simulink model "BD_HESS_K"  (R2024b)
settings: Solver=ode1  StartTime=0.0  StopTime=1369  FixedStep=0.1  MaxStep=1  RelTol=1e-3  AbsTol=1e-3
values from neighbouring files (symbols this model uses):
  ess2_cap = [ ... (first row only)    [ESS2_SC_MaxwellBCAP3400F.m]
  ess2_cap_scale = 1    [ESS2_SC_MaxwellBCAP3400F.m]
  ess2_coulombic_eff = [ ... (first row only)    [ESS2_SC_MaxwellBCAP3400F.m]
  ess2_init_soc = 1    [ESS2_SC_MaxwellBCAP3400F.m]
  ess2_max_volts = 2.7*120    (= 324)    [ESS2_SC_MaxwellBCAP3400F.m]
  ess2_min_volts = 0*2.7*120    (= 0)    [ESS2_SC_MaxwellBCAP3400F.m]
  ess2_mod_init_tmp = 20    [ESS2_SC_MaxwellBCAP3400F.m]
  ess2_module_num = 1    [ESS2_SC_MaxwellBCAP3400F.m]
  ess2_parallel_mod_num = 1    [ESS2_SC_MaxwellBCAP3400F.m]
  ess2_r = [ ... (first row only)    [ESS2_SC_MaxwellBCAP3400F.m]
  ess2_res_scale_coef = [1 0 1 0]    [ESS2_SC_MaxwellBCAP3400F.m]
  ess2_res_scale_fun = inline('(x(1)*ess2_module_num+x(2))/(x(3)*ess2_cap_scale+x(4))','x','ess2_module_num','ess2_cap_scale')    [ESS2_SC_MaxwellBCAP3400F.m]
  ess2_tmp = [-20 -10 0 5 10 15 20 25 30 40 50 60 65]    [ESS2_SC_MaxwellBCAP3400F.m]
  ess_cap_scale = 1    [ESS_Panasonic_NCR18650B_params.m]
  ess_coulombic_eff = [0.863 0.957 0.959 0.967 0.994]    [ESS_Panasonic_NCR18650B_params.m]
  ess_init_soc = 1    [ESS_Panasonic_NCR18650B_params.m]
  ess_max_ah_cap = [2.78 2.92 3.09 3.27 3.31]*74    [ESS_Panasonic_NCR18650B_params.m]
  ess_max_volts = 4.2*6    (= 25.2)    [ESS_Panasonic_NCR18650B_params.m]
  ess_min_volts = 2.5*6    (= 15)    [ESS_Panasonic_NCR18650B_params.m]
  ess_mod_init_tmp = 20    [ESS_Panasonic_NCR18650B_params.m]
  ess_module_num = 16    [ESS_Panasonic_NCR18650B_params.m]
  ess_on = 1    [ESS_Panasonic_NCR18650B_params.m]
  ess_r_chg = [0.0470 0.0457 0.0448 0.0435 0.0429 0.0427 0.0429 0.0462 ... (first row only)    [ESS_Panasonic_NCR18650B_params.m]
  ess_r_dis = [0.0470 0.0457 0.0448 0.0435 0.0429 0.0427 0.0429 0.0462 ... (first row only)    [ESS_Panasonic_NCR18650B_params.m]
  ess_res_scale_coef = [1 0 1 0]    [ESS_Panasonic_NCR18650B_params.m]
  ess_res_scale_fun = inline('(x(1)*ess_module_num+x(2))/(x(3)*ess_cap_scale+x(4))','x','ess_module_num','ess_cap_scale')    [ESS_Panasonic_NCR18650B_params.m]
  ess_soc = [0 10 20 40 60 80 90 100]/100    [ESS_Panasonic_NCR18650B_params.m]
  ess_tmp = [-10 0 10 25 45]    [ESS_Panasonic_NCR18650B_params.m]
  ess_voc = [2.5 2.74 2.93 3.17 3.36 3.5 3.49 3.34 ... (first row only)    [ESS_Panasonic_NCR18650B_params.m]
  mc_min_volts = 0    [ESS_Panasonic_NCR18650B_params.m]
  pth = pth_values(i)    [Ems_code_for_set_EMSvalue.m]
undefined symbols (not defined in the file or in its folder): power_load_in_Watt
(part 1 of 2)
settings Model: ModifiedComment=45089 -- Tue Apr 22 21:30:29 2025 -- Version 24.2  Creator=mokeefe  LastModifiedBy=ZULFI
settings Model: ModifiedHistory=|
  | 45089 -- Tue Apr 22 21:30:29 2025 -- Version 24.2
  | 
  | 45089 -- Tue Apr 22 21:18:21 2025 -- Version 24.1
  | 
  | 45089 -- Tue Apr 22 18:42:21 2025 -- Version 24.0
  | 
  | HP -- Sat Sep 19 16:11:01 2020 -- Version 1.240
  | 
  | 
  | HP -- Sat Sep 19 16:09:55 2020 -- Version 1.239
  | 
  | 
  | tz1n17 -- Sat Mar 30 21:57:00 2019 -- Version 1.238
  | 
  | 
  | tz1n17 -- Sat Mar 30 21:36:30 2019 -- Version 1.237
  | 
  | 
  | tz1n17 -- Sat Mar 30 21:35:16 2019 -- Version 1.236
  | 
  | 
  | tz1n17 -- Wed Mar 06 15:26:13 2019 -- Version 1.235
  | 
  | 
  | tz1n17 -- Wed Mar 06 15:22:09 2019 -- Version 1.234
  | 
  | 
  | tz1n17 -- Wed Mar 06 15:20:42 2019 -- Version 1.233
  | 
  | 
  | tz1n17 -- Wed Mar 06 15:19:06 2019 -- Version 1.232
  | 
  | 
  | tz1n17 -- Wed Mar 06 15:00:51 2019 -- Version 1.231
  | 
  | 
  | tz1n17 -- Wed Mar 06 14:47:09 2019 -- Version 1.230
  | 
  | 
  | tz1n17 -- Wed Mar 06 14:46:20 2019 -- Version 1.229
  | 
  | 
  | tz1n17 -- Wed Mar 06 14:42:10 2019 -- Version 1.228
  | 
  | 
  | tz1n17 -- Wed Mar 06 14:36:58 2019 -- Version 1.227
  | 
  | 
  | tz1n17 -- Wed Mar 06 13:46:14 2019 -- Version 1.226
  | 
  | 
  | tz1n17 -- Wed Mar 06 13:45:11 2019 -- Version 1.225
  | 
  | 
  | tz1n17 -- Wed Mar 06 12:23:18 2019 -- Version 1.224
  | 
  | 
  | tz1n17 -- Tue Mar 05 16:46:13 2019 -- Version 1.223
  | 
  | 
  | tz1n17 -- Tue Mar 05 16:36:09 2019 -- Version 1.222
  | 
  | 
  | tz1n17 -- Tue Mar 05 16:31:19 2019 -- Version 1.221
  | 
  | 
  | tz1n17 -- Tue Mar 05 15:30:42 2019 -- Version 1.220
  | 
  | 
  | tz1n17 -- Tue Mar 05 15:29:22 2019 -- Version 1.219
  | 
  | 
  | tz1n17 -- Tue Mar 05 15:24:15 2019 -- Version 1.218
  | 
  | 
  | tz1n17 -- Tue Mar 05 15:23:28 2019 -- Version 1.217
  | 
  | 
  | tz1n17 -- Tue Mar 05 15:23:21 2019 -- Version 1.216
  | 
  | 
  | tz1n17 -- Tue Mar 05 15:16:39 2019 -- Version 1.215
  | 
  | 
  | tz1n17 -- Tue Mar 05 15:14:45 2019 -- Version 1.214
  | 
  | 
  | tz1n17 -- Tue Mar 05 15:13:01 2019 -- Version 1.213
  | 
  | 
  | tz1n17 -- Tue Mar 05 15:09:24 2019 -- Version 1.212
  | 
  | 
  | tz1n17 -- Tue Mar 05 15:02:33 2019 -- Version 1.211
  | 
  | 
  | tz1n17 -- Tue Mar 05 15:01:02 2019 -- Version 1.210
  | 
  | 
  | tz1n17 -- Mon Mar 04 22:33:33 2019 -- Version 1.209
  | 
  | 
  | tz1n17 -- Mon Mar 04 22:09:23 2019 -- Version 1.208
  | 
  | 
  | tz1n17 -- Mon Mar 04 21:44:15 2019 -- Version 1.207
  | 
  | 
  | tz1n17 -- Mon Mar 04 21:41:50 2019 -- Version 1.206
  | 
  | 
  | tz1n17 -- Mon Mar 04 21:41:07 2019 -- Version 1.205
  | 
  | 
  | HP -- Mon Mar 04 01:45:44 2019 -- Version 1.204
  | 
  | 
  | HP -- Mon Mar 04 01:39:57 2019 -- Version 1.203
  | 
  | 
  | HP -- Mon Mar 04 01:37:38 2019 -- Version 1.202
  | 
  | 
  | HP -- Mon Mar 04 01:08:49 2019 -- Version 1.201
  | 
  | 
  | HP -- Mon Mar 04 01:02:45 2019 -- Version 1.200
  | 
  | 
  | HP -- Mon Mar 04 00:48:56 2019 -- Version 1.199
  | 
  | 
  | tz1n17 -- Sun Mar 03 22:48:13 2019 -- Version 1.198
  | 
  | 
  | tz1n17 -- Sun Mar 03 22:46:29 2019 -- Version 1.197
  | 
  | 
  | tz1n17 -- Sun Mar 03 21:57:47 2019 -- Version 1.196
  | 
  | 
  | tz1n17 -- Sun Mar 03 21:10:24 2019 -- Version 1.195
  | 
  | 
  | tz1n17 -- Sun Mar 03 21:06:11 2019 -- Version 1.194
  | 
  | 
  | tz1n17 -- Sun Mar 03 20:55:37 2019 -- Version 1.193
  | 
  | 
  | tz1n17 -- Sun Mar 03 20:49:58 2019 -- Version 1.192
  | 
  | 
  | tz1n17 -- Mon Feb 25 15:47:07 2019 -- Version 1.191
  | 
  | 
  | tz1n17 -- Mon Feb 25 15:37:36 2019 -- Version 1.190
  | 
  | 
  | tz1n17 -- Mon Feb 25 14:55:26 2019 -- Version 1.189
  | 
  | 
  | tz1n17 -- Mon Feb 25 14:54:22 2019 -- Version 1.188
  | 
  | 
  | tz1n17 -- Mon Feb 25 14:54:08 2019 -- Version 1.187
  | 
  | 
  | tz1n17 -- Fri Feb 15 22:56:00 2019 -- Version 1.186
  | 
  | 
  | tz1n17 -- Wed Dec 19 14:48:50 2018 -- Version 1.185
  | 
  | 
  | tz1n17 -- Tue Dec 18 22:44:41 2018 -- Version 1.184
  | 
  | 
  | tz1n17 -- Tue Dec 18 18:15:37 2018 -- Version 1.183
  | 
  | 
  | tz1n17 -- Tue Dec 18 18:08:38 2018 -- Version 1.182
  | 
  | 
  | tz1n17 -- Tue Dec 18 17:38:08 2018 -- Version 1.181
  | 
  | 
  | tz1n17 -- Mon Dec 17 22:41:01 2018 -- Version 1.180
  | 
  | 
  | tz1n17 -- Mon Dec 17 20:34:34 2018 -- Version 1.179
  | 
  | 
  | tz1n17 -- Mon Dec 17 17:22:02 2018 -- Version 1.178
  | 
  | 
  | tz1n17 -- Wed Dec 12 22:54:23 2018 -- Version 1.177
  | 
  | 
  | tz1n17 -- Wed Dec 12 20:45:31 2018 -- Version 1.176
  | 
  | 
  | tz1n17 -- Tue Dec 11 15:05:18 2018 -- Version 1.175
  | 
  | 
  | tz1n17 -- Tue Dec 11 14:54:48 2018 -- Version 1.174
  | 
  | 
  | tz1n17 -- Tue Dec 11 14:50:01 2018 -- Version 1.173
  | 
  | 
  | tz1n17 -- Tue Dec 11 14:47:20 2018 -- Version 1.172
  | 
  | 
  | tz1n17 -- Tue Dec 11 14:46:21 2018 -- Version 1.171
  | 
  | 
  | tz1n17 -- Tue Dec 11 14:36:41 2018 -- Version 1.170
  | 
  | 
  | tz1n17 -- Tue Dec 11 14:22:13 2018 -- Version 1.169
  | 
  | 
  | tz1n17 -- Tue Dec 11 14:20:14 2018 -- Version 1.168
  | 
  | 
  | tz1n17 -- Sun Dec 09 22:34:26 2018 -- Version 1.167
  | 
  | 
  | tz1n17 -- Sun Dec 09 22:33:45 2018 -- Version 1.166
  | 
  | 
  | tz1n17 -- Sun Dec 09 22:25:11 2018 -- Version 1.165
  | 
  | 
  | tz1n17 -- Sun Dec 09 22:23:19 2018 -- Version 1.164
  | 
  | 
  | tz1n17 -- Sun Dec 09 22:22:45 2018 -- Version 1.163
  | 
  | 
  | tz1n17 -- Sun Dec 09 22:21:43 2018 -- Version 1.162
  | 
  | 
  | tz1n17 -- Sun Dec 09 22:20:11 2018 -- Version 1.161
  | 
  | 
  | tz1n17 -- Sun Dec 09 22:19:52 2018 -- Version 1.160
  | 
  | 
  | tz1n17 -- Sun Dec 09 22:01:56 2018 -- Version 1.159
  | 
  | 
  | tz1n17 -- Sun Dec 09 21:58:21 2018 -- Version 1.158
  | 
  | 
  | tz1n17 -- Sun Dec 09 21:55:12 2018 -- Version 1.157
  | 
  | 
  | tz1n17 -- Sun Dec 09 21:51:49 2018 -- Version 1.156
  | 
  | 
  | tz1n17 -- Sun Dec 09 21:49:03 2018 -- Version 1.155
  | 
  | 
  | tz1n17 -- Sun Dec 09 21:48:14 2018 -- Version 1.154
  | 
  | 
  | tz1n17 -- Sun Dec 09 21:32:48 2018 -- Version 1.153
  | 
  | 
  | tz1n17 -- Sun Dec 09 20:07:47 2018 -- Version 1.152
  | 
  | 
  | tz1n17 -- Sun Dec 09 18:47:48 2018 -- Version 1.151
  | 
  | 
  | tz1n17 -- Sun Dec 09 18:18:43 2018 -- Version 1.150
  | 
  | 
  | HP -- Sun Dec 09 02:13:19 2018 -- Version 1.149
  | 
  | 
  | tz1n17 -- Sat Dec 08 22:45:48 2018 -- Version 1.148
  | 
  | 
  | tz1n17 -- Sat Dec 08 18:27:05 2018 -- Version 1.147
  | 
  | 
  | HP -- Sat Dec 08 00:10:24 2018 -- Version 1.146
  | 
  | 
  | HP -- Sat Dec 08 00:03:06 2018 -- Version 1.145
  | 
  | 
  | HP -- Fri Dec 07 23:56:35 2018 -- Version 1.144
  | 
  | 
  | tz1n17 -- Fri Dec 07 22:43:57 2018 -- Version 1.143
  | 
  | 
  | tz1n17 -- Fri Dec 07 22:21:30 2018 -- Version 1.142
  | 
  | 
  | tz1n17 -- Fri Dec 07 21:44:41 2018 -- Version 1.141
  | 
  | 
  | tz1n17 -- Fri Dec 07 21:41:03 2018 -- Version 1.140
  | 
  | 
  | tz1n17 -- Fri Dec 07 21:39:48 2018 -- Version 1.139
  | 
  | 
  | tz1n17 -- Fri Dec 07 18:02:33 2018 -- Version 1.138
  | 
  | 
  | tz1n17 -- Fri Dec 07 17:48:39 2018 -- Version 1.137
  | 
  | 
  | tz1n17 -- Fri Dec 07 15:16:04 2018 -- Version 1.136
  | 
  | 
  | tz1n17 -- Fri Dec 07 15:05:37 2018 -- Version 1.135
  | 
  | 
  | tz1n17 -- Fri Dec 07 14:56:20 2018 -- Version 1.134
  | 
  | 
  | tz1n17 -- Fri Dec 07 13:49:20 2018 -- Version 1.133
  | 
  | 
  | tz1n17 -- Fri Dec 07 13:47:15 2018 -- Version 1.132
  | 
  | 
  | tz1n17 -- Thu Dec 06 15:55:35 2018 -- Version 1.131
  | 
  | 
  | tz1n17 -- Thu Dec 06 15:03:27 2018 -- Version 1.130
  | 
  | 
  | tz1n17 -- Tue Dec 04 17:57:34 2018 -- Version 1.129
  | 
  | 
  | tz1n17 -- Tue Dec 04 15:03:13 2018 -- Version 1.128
  | 
  | 
  | tz1n17 -- Tue Dec 04 14:53:19 2018 -- Version 1.127
  | 
  | 
  | tz1n17 -- Tue Dec 04 14:45:06 2018 -- Version 1.126
  | 
  | 
  | tz1n17 -- Tue Dec 04 14:39:30 2018 -- Version 1.125
  | 
  | 
  | tz1n17 -- Tue Dec 04 14:29:06 2018 -- Version 1.124
  | 
  | 
  | HP -- Sun Dec 02 02:48:45 2018 -- Version 1.123
  | 
  | 
  | HP -- Sun Dec 02 01:47:26 2018 -- Version 1.122
  | 
  | 
  | HP -- Sun Dec 02 01:13:09 2018 -- Version 1.121
  | 
  | 
  | tz1n17 -- Sat Dec 01 23:02:41 2018 -- Version 1.120
  | 
  | 
  | tz1n17 -- Sat Dec 01 23:01:08 2018 -- Version 1.119
  | 
  | 
  | tz1n17 -- Sat Dec 01 22:57:45 2018 -- Version 1.118
  | 
  | 
  | tz1n17 -- Wed Nov 28 20:22:41 2018 -- Version 1.117
  | 
  | 
  | tz1n17 -- Wed Nov 28 20:01:59 2018 -- Version 1.116
  | 
  | 
  | tz1n17 -- Wed Nov 28 20:00:05 2018 -- Version 1.115
  | 
  | 
  | tz1n17 -- Wed Nov 28 19:59:42 2018 -- Version 1.114
  | 
  | 
  | tz1n17 -- Wed Nov 28 19:39:22 2018 -- Version 1.113
  | 
  | 
  | tz1n17 -- Wed Nov 28 19:29:55 2018 -- Version 1.112
  | 
  | 
  | tz1n17 -- Wed Nov 28 19:29:15 2018 -- Version 1.111
  | 
  | 
  | tz1n17 -- Wed Nov 28 19:28:44 2018 -- Version 1.110
  | 
  | 
  | tz1n17 -- Wed Nov 28 19:26:40 2018 -- Version 1.109
  | 
  | 
  | tz1n17 -- Wed Nov 28 19:25:31 2018 -- Version 1.108
  | 
  | 
  | tz1n17 -- Wed Nov 28 19:24:33 2018 -- Version 1.107
  | 
  | 
  | tz1n17 -- Wed Nov 28 19:15:20 2018 -- Version 1.106
  | 
  | 
  | tz1n17 -- Wed Nov 28 19:13:31 2018 -- Version 1.105
  | 
  | 
  | tz1n17 -- Wed Nov 28 19:11:29 2018 -- Version 1.103
  | 
  | 
  | tz1n17 -- Wed Nov 28 19:12:22 2018 -- Version 1.103
  | 
  | 
  | tz1n17 -- Wed Nov 28 19:08:22 2018 -- Version 1.102
  | 
  | 
  | tz1n17 -- Wed Nov 28 19:03:07 2018 -- Version 1.101
  | 
  | 
  | tz1n17 -- Wed Nov 28 18:47:53 2018 -- Version 1.100
  | 
  | 
  | tz1n17 -- Wed Nov 28 18:45:05 2018 -- Version 1.99
  | 
  | 
  | tz1n17 -- Wed Nov 28 18:29:30 2018 -- Version 1.98
  | 
  | 
  | tz1n17 -- Wed Nov 28 18:02:53 2018 -- Version 1.97
  | 
  | 
  | tz1n17 -- Wed Nov 28 18:01:36 2018 -- Version 1.96
  | 
  | 
  | tz1n17 -- Wed Nov 28 17:50:17 2018 -- Version 1.95
  | 
  | 
  | tz1n17 -- Wed Nov 28 17:44:30 2018 -- Version 1.94
  | 
  | 
  | tz1n17 -- Wed Nov 28 17:38:14 2018 -- Version 1.93
  | 
  | 
  | tz1n17 -- Wed Nov 28 15:16:29 2018 -- Version 1.92
  | 
  | 
  | tz1n17 -- Wed Nov 28 15:15:00 2018 -- Version 1.91
  | 
  | 
  | tz1n17 -- Wed Nov 28 15:13:10 2018 -- Version 1.90
  | 
  | 
  | tz1n17 -- Wed Nov 28 15:12:41 2018 -- Version 1.89
  | 
  | 
  | tz1n17 -- Wed Nov 28 15:10:02 2018 -- Version 1.88
  | 
  | 
  | tz1n17 -- Wed Nov 28 15:05:39 2018 -- Version 1.87
  | 
  | 
  | tz1n17 -- Wed Nov 28 15:05:01 2018 -- Version 1.86
  | 
  | 
  | tz1n17 -- Wed Nov 28 14:59:02 2018 -- Version 1.85
  | 
  | 
  | tz1n17 -- Wed Nov 28 14:58:38 2018 -- Version 1.84
  | 
  | 
  | tz1n17 -- Wed Nov 28 14:57:57 2018 -- Version 1.83
  | 
  | 
  | tz1n17 -- Wed Nov 28 14:56:25 2018 -- Version 1.82
  | 
  | 
  | tz1n17 -- Wed Nov 28 14:55:58 2018 -- Version 1.81
  | 
  | 
  | tz1n17 -- Wed Nov 28 14:54:44 2018 -- Version 1.80
  | 
  | 
  | tz1n17 -- Wed Nov 28 14:52:16 2018 -- Version 1.79
  | 
  | 
  | tz1n17 -- Wed Nov 28 14:50:51 2018 -- Version 1.78
  | 
  | 
  | tz1n17 -- Wed Nov 28 14:50:00 2018 -- Version 1.77
  | 
  | 
  | tz1n17 -- Wed Nov 28 14:45:14 2018 -- Version 1.76
  | 
  | 
  | tz1n17 -- Wed Nov 28 14:33:34 2018 -- Version 1.75
  | 
  | 
  | tz1n17 -- Wed Nov 28 13:43:19 2018 -- Version 1.74
  | 
  | 
  | tz1n17 -- Tue Nov 27 23:20:40 2018 -- Version 1.73
  | 
  | 
  | tz1n17 -- Tue Nov 27 23:12:46 2018 -- Version 1.72
  | 
  | 
  | tz1n17 -- Tue Nov 27 23:10:27 2018 -- Version 1.71
  | 
  | 
  | tz1n17 -- Tue Nov 27 20:21:58 2018 -- Version 1.70
  | 
  | 
  | tz1n17 -- Tue Nov 27 20:17:34 2018 -- Version 1.69
  | 
  | 
  | tz1n17 -- Tue Nov 27 20:09:17 2018 -- Version 1.68
  | 
  | 
  | tz1n17 -- Tue Nov 27 20:06:13 2018 -- Version 1.67
  | 
  | 
  | tz1n17 -- Tue Nov 27 19:10:28 2018 -- Version 1.66
  | 
  | 
  | tz1n17 -- Tue Nov 27 18:48:36 2018 -- Version 1.65
  | 
  | 
  | tz1n17 -- Tue Nov 27 18:42:18 2018 -- Version 1.64
  | 
  | 
  | tz1n17 -- Tue Nov 27 18:22:46 2018 -- Version 1.63
  | 
  | 
  | tz1n17 -- Tue Nov 27 18:11:41 2018 -- Version 1.62
  | 
  | 
  | tz1n17 -- Tue Nov 27 17:00:22 2018 -- Version 1.61
  | 
  | 
  | tz1n17 -- Tue Nov 27 16:46:06 2018 -- Version 1.60
  | 
  | 
  | tz1n17 -- Tue Nov 27 16:40:59 2018 -- Version 1.59
  | 
  | 
  | tz1n17 -- Tue Nov 27 14:28:49 2018 -- Version 1.58
  | 
  | 
  | tz1n17 -- Tue Nov 27 14:23:14 2018 -- Version 1.57
  | 
  | 
  | tz1n17 -- Tue Nov 27 14:01:43 2018 -- Version 1.56
  | 
  | 
  | tz1n17 -- Tue Nov 27 14:01:03 2018 -- Version 1.55
  | 
  | 
  | tz1n17 -- Tue Nov 27 13:50:04 2018 -- Version 1.54
  | 
  | 
  | tz1n17 -- Tue Nov 27 13:39:43 2018 -- Version 1.53
  | 
  | 
  | tz1n17 -- Mon Nov 26 22:49:44 2018 -- Version 1.52
  | 
  | 
  | tz1n17 -- Mon Nov 26 21:02:43 2018 -- Version 1.51
  | 
  | 
  | tz1n17 -- Mon Nov 26 20:38:16 2018 -- Version 1.50
  | 
  | 
  | tz1n17 -- Mon Nov 26 14:59:15 2018 -- Version 1.49
  | 
  | 
  | tz1n17 -- Mon Nov 26 14:25:02 2018 -- Version 1.48
  | 
  | 
  | tz1n17 -- Sun Nov 25 17:04:50 2018 -- Version 1.47
  | 
  | 
  | tz1n17 -- Sun Nov 25 16:33:53 2018 -- Version 1.46
  | 
  | 
  | tz1n17 -- Sat Nov 24 23:14:29 2018 -- Version 1.45
  | 
  | 
  | tz1n17 -- Wed Nov 21 22:02:06 2018 -- Version 1.44
  | 
  | 
  | tz1n17 -- Mon Oct 29 23:01:38 2018 -- Version 1.43
  | 
  | 
  | tz1n17 -- Mon Oct 29 22:46:10 2018 -- Version 1.42
  | 
  | 
  | tz1n17 -- Mon Oct 29 22:41:06 2018 -- Version 1.41
  | 
  | 
  | tz1n17 -- Mon Oct 29 22:23:29 2018 -- Version 1.40
  | 
  | 
  | tz1n17 -- Mon Oct 29 16:17:50 2018 -- Version 1.39
  | 
  | 
  | mokeefe -- Fri Mar 23 15:18:43 2012 -- Version 1.38
  | Updated parameterized link to restore library link. Save to update to newset Simulink version.
  | 
  | ssprik -- Wed Sep 24 14:52:29 2003 -- Version 1.37
  | 
  | 
  | abrooker -- Tue May 14 11:43:34 2002 -- Version 1.36
  | 
  | 
  | mokeefe -- Thu Apr 18 07:55:22 2002 -- Version 1.35
  | saving the model:
  | o "without the model browser open"
  | o with only top-level screen visible
  | o and with "fit to view" enabled
  | 
  | mokeefe -- Thu Apr 18 07:44:56 2002 -- Version 1.34
  | saving the model:
  | o "without the model browser open"
  | o with only top-level screen visible
  | o and with "fit to view" enabled
settings SolverCC: AutoScaleAbsTol=off  AlgebraicLoopSolver=TrustRegion
settings DataIOCC: SaveFormat=Array  SignalLoggingSaveFormat=ModelDataLogs  SaveOutput=off  SaveTime=off  ReturnWorkspaceOutputs=off
settings OptimizationCC: BooleanDataType=off  ExpressionDepthLimit=2147483647  LifeSpan=inf
settings DebuggingCC: SaveWithParameterizedLinksMsg=none  UnderspecifiedInitializationDetection=Classic  MergeDetectMultiDrivingBlocksExec=none  SignalResolutionControl=TryResolveAllWithWarning  MultiTaskDSMMsg=warning  MultiTaskCondExecSysMsg=none  FcnCallInpInsideContextMsg=warning  UnconnectedInputMsg=warning  UnconnectedOutputMsg=warning  StateNameClashWarn=warning  SFUnexpectedBacktrackingDiag=warning  SFNoUnconditionalDefaultTransitionDiag=warning  SFExecutionAtInitializationDiag=none  ArithmeticOperatorsInVariantConditions=warning
settings HardwareCC: ProdBitPerPointer=32  ProdBitPerSizeT=32  ProdBitPerPtrDiffT=32  ProdLargestAtomicFloat=None  ProdIntDivRoundTo=Undefined  ProdEndianess=Unspecified  ProdWordSize=32  ProdHWDeviceType=32-bit Generic  TargetUnknown=on
settings ModelReferenceCC: PropagateSignalLabelsOutOfModel=off
settings SFSimCC: SimUseLocalCustomCode=off  CustomCodeUndefinedFunction=UseInterfaceOnly
settings RTWCC: TemplateMakefile=grt_vc.tmf  RTWUseLocalCustomCode=off  GPUComputeCapability=3.5
settings CodeAppCC: StateflowObjectComments=on
settings GRTTargetCC: TargetLangStandard=C89/C90 (ANSI)  CombineOutputUpdateFcns=off  GRTInterface=on
settings ConfigComp: CovMetricSettings=dw  CovSaveCumulativeToWorkspaceVar=on  CovSaveSingleToWorkspaceVar=on  CovExternalEMLEnable=off

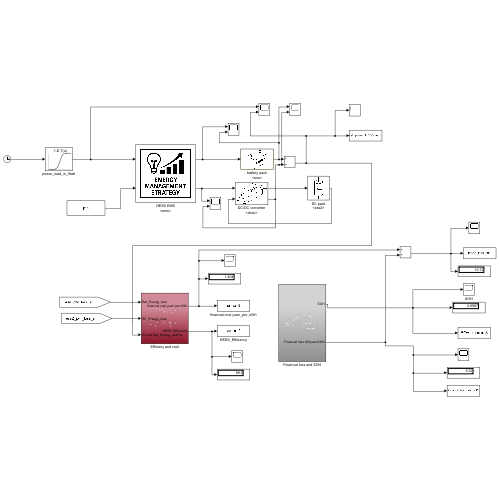
[thumbnail: Simulink's stored preview of the top-level diagram]
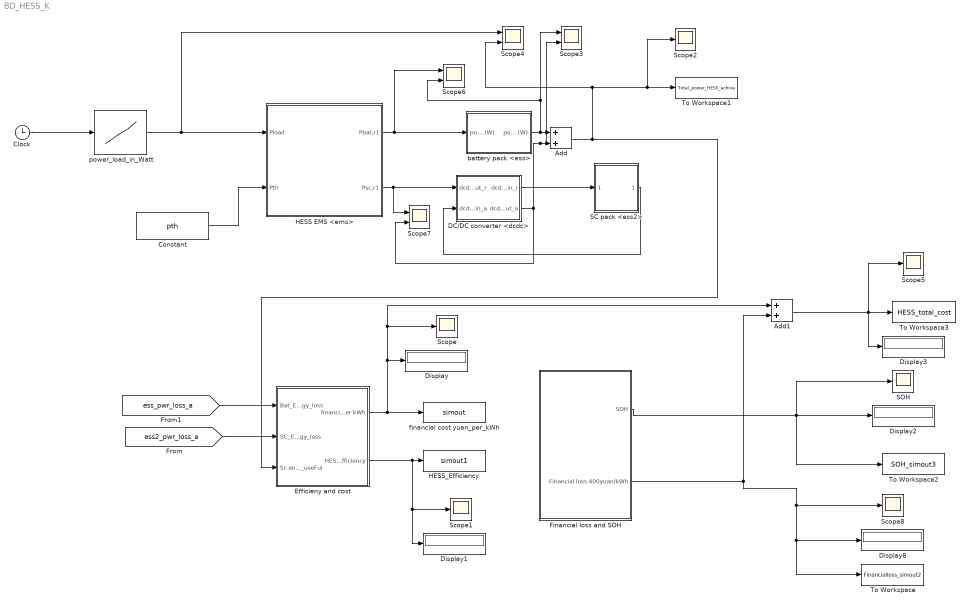
== system BD_HESS_K ==
  Add : Sum
  Add1 : Sum
  Clock : Clock
      settings: Decimation=1369
  Constant : Constant  Value=pth
  "DC/DC converter <dcdc> " : Subsystem  AncestorBlock=|
      | lib_energy_storage/Ess Choices/DC//DC <dcdc>
      | Eff model 
      | without electrical presentations
      mask Display: image('Image21_27_51.png');
  Display{,1..3,8} (5 alike) : Display
  Efficieny and cost : Subsystem
  Financial loss and SOH : Subsystem
  HESS EMS <ems> : Subsystem  AncestorBlock=|
      | lib_controls/HESS Control Strategy
      | <ems>
      | Logic Threshold (BAT) CS2
      mask Display: image(['Image22_01_33.png'])
  HESS_Efficiency : ToWorkspace  VariableName=simout1  SaveFormat=Timeseries  SampleTime=-1
  "SC pack <ess2> " : Subsystem  AncestorBlock=|
      | lib_energy_storage/Ess Choices/Ultracapacitor
      |  System
      | <uc>
      | CapLoss&Cost
      mask Display: image('Image21_26_34.png');
  SOH : Scope
  Scope{,1..2,5,8} (5 alike) : Scope
  Scope{3..4,6..7} (4 alike) : Scope  NumInputPorts=2
  To Workspace : ToWorkspace  VariableName=Financialloss_simout2  SaveFormat=Timeseries  SampleTime=-1
  To Workspace1 : ToWorkspace  VariableName=Total_power_HESS_achive  SaveFormat=Timeseries  SampleTime=-1
  To Workspace2 : ToWorkspace  VariableName=SOH_simout3  SaveFormat=Timeseries  SampleTime=-1
  To Workspace3 : ToWorkspace  VariableName=HESS_total_cost  SaveFormat=Timeseries  SampleTime=-1
  battery pack <ess> : Subsystem  AncestorBlock=|
      | lib_energy_storage/Ess Choices/energy
      | storage <ess>
      | CapLoss Modified
      mask Display: image('Image21_26_45.png');
  financial cost yuan_per_kWh : ToWorkspace  VariableName=simout  SaveFormat=Timeseries  SampleTime=-1
  power_load_in_Watt : Lookup_n-D  NumberOfTableDimensions=1  BreakpointsForDimension1=0:1369  Table=power_load_in_Watt  InternalRulePriority=Speed  RndMeth=Simplest
  wires:
  battery pack <ess>/1(power available to bus (W)) -> Scope6/2, Scope3/1, Add/1
  Add/1 -> Efficieny and cost/3(Sc and Bat_Energy_useFul), Scope2/1, To Workspace1/1, Scope4/2
  "DC/DC converter <dcdc> "/1(" dcdc_power_in_r ") -> "SC pack <ess2> "/1(power req'd into bus (W))
  HESS EMS <ems>/2(Psc,r1) -> Scope7/1, "DC/DC converter <dcdc> "/1(dcdc_power_out_r)
  HESS EMS <ems>/1(Pbat,r1) -> Scope6/1, battery pack <ess>/1(power req'd into bus (W))
  "SC pack <ess2> "/1(power available to bus (W)) -> "DC/DC converter <dcdc> "/2(dcdc_power_in_a)
  Clock/1 -> power_load_in_Watt/1
  Efficieny and cost/2(HESS_Efficiency) -> Display1/1, Scope1/1, HESS_Efficiency/1
  Efficieny and cost/1(" financial cost yuan per kWh") -> Add1/1, Scope/1, Display/1, financial cost yuan_per_kWh/1
  [ess2_pwr_loss_a] -> Efficieny and cost/2(SC_Energy_loss)
  [ess_pwr_loss_a] -> Efficieny and cost/1("Bat_Energy_loss ")
  Financial loss and SOH/1(SOH) -> SOH/1, To Workspace2/1, Display2/1
  Financial loss and SOH/2(Financial loss 400yuan/kWh) -> To Workspace/1, Display8/1, Scope8/1, Add1/2
  Add1/1 -> Display3/1, Scope5/1, To Workspace3/1
  Constant/1 -> HESS EMS <ems>/2(Pth)
  "DC/DC converter <dcdc> "/2(" dcdc_power_out_a") -> Scope3/2, Add/2, Scope7/2
  power_load_in_Watt/1 -> HESS EMS <ems>/1(Pload), Scope4/1

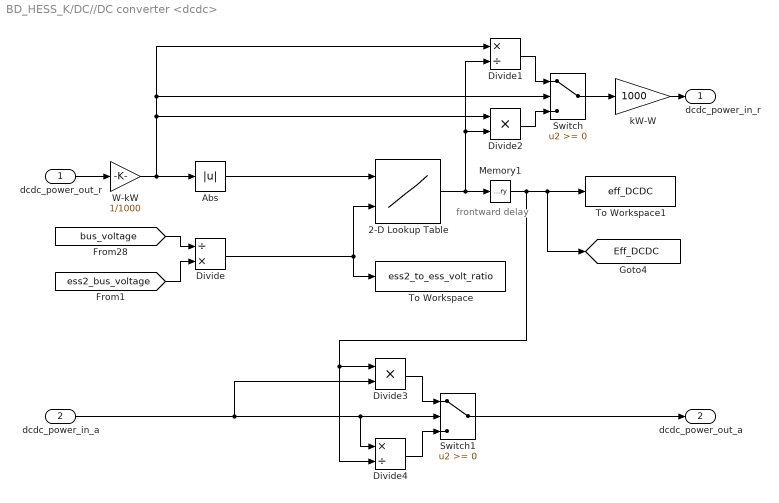
== system BD_HESS_K/DC//DC converter <dcdc>  ==
  note: frontward delay
  dcdc_power_out_r : Inport
  dcdc_power_in_a : Inport  Port=2
  2-D Lookup Table : Lookup_n-D  BreakpointsForDimension1=[0,20,40,60,80,360]  BreakpointsForDimension2=[0,0.2,0.4,0.6,0.8,1]  Table=reshape([0.8,0.945,0.94,0.938,0.934,0.934,0.8,0.945,0.94,0.938,0.934,0.934,0.8,0.952,0.95,0.946,0.944,0.944,0.8,0.965,0.957,0.952,0.95,0.95,0.8,0.972,0.965,0.962,0.96,0.96,0.8,0.977,0.97,0.964,0.962,0.962],6,6)  RndMeth=Simplest
      settings: InputPortMap=u0,u1
  Abs : Abs  SaturateOnIntegerOverflow=off
  Divide : Product  Inputs=/*
  Divide1 : Product  Inputs=*/
  Divide2 : Product  Inputs=**
  Divide3 : Product  Inputs=**
  Divide4 : Product  Inputs=*/
  Memory1 : Memory  InitialCondition=0.95
  Switch : Switch  SaturateOnIntegerOverflow=off  InputSameDT=off
  Switch1 : Switch  SaturateOnIntegerOverflow=off  InputSameDT=off
  To Workspace : ToWorkspace  VariableName=ess2_to_ess_volt_ratio  SaveFormat=Timeseries  SampleTime=-1
  To Workspace1 : ToWorkspace  VariableName=eff_DCDC  SaveFormat=Timeseries  SampleTime=-1
  W-kW : Gain  Gain=1/1000
  kW-W : Gain  Gain=1000
  " dcdc_power_in_r " : Outport
  " dcdc_power_out_a" : Outport  Port=2
  tag scope: Eff_DCDC=global
  wires:
  Divide4/1 -> Switch1/3
  Divide3/1 -> Switch1/1
  dcdc_power_in_a/1 -> Switch1/2, Divide4/1, Divide3/2
  kW-W/1 -> " dcdc_power_in_r "/1
  W-kW/1 -> Abs/1, Switch/2, Divide1/1, Divide2/1
  Switch/1 -> kW-W/1
  Divide2/1 -> Switch/3
  Divide1/1 -> Switch/1
  Divide/1 -> To Workspace/1, 2-D Lookup Table/2
  dcdc_power_out_r/1 -> W-kW/1
  [bus_voltage] -> Divide/1
  [ess2_bus_voltage] -> Divide/2
  Switch1/1 -> " dcdc_power_out_a"/1
  2-D Lookup Table/1 -> Memory1/1, Divide1/2, Divide2/2
  Abs/1 -> 2-D Lookup Table/1
  Memory1/1 -> Divide4/2, Divide3/1, [Eff_DCDC], To Workspace1/1

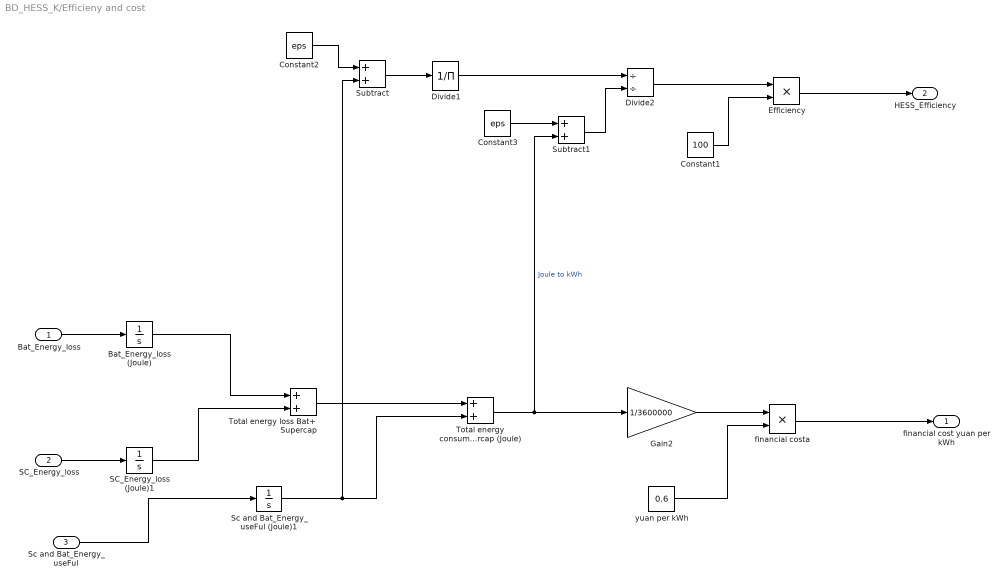
== system BD_HESS_K/Efficieny and cost ==
  "Bat_Energy_loss " : Inport
  SC_Energy_loss : Inport  Port=2
  Sc and Bat_Energy_useFul : Inport  Port=3
  Bat_Energy_loss (Joule) : Integrator
  Constant1 : Constant  Value=100
  Constant2 : Constant  Value=eps
  Constant3 : Constant  Value=eps
  Divide1 : Product  Inputs=/
  Divide2 : Product  Inputs=//
  Efficiency : Product
  Gain2 : Gain  Gain=1/3600000
  SC_Energy_loss (Joule)1 : Integrator
  Sc and Bat_Energy_useFul (Joule)1 : Integrator
  Subtract : Sum
  Subtract1 : Sum
  Total energy consumption Bat+ Supercap (Joule) : Sum
  Total energy loss Bat+ Supercap : Sum
  financial costa : Product
  yuan per kWh : Constant  Value=0.6
  " financial cost yuan per kWh" : Outport
  HESS_Efficiency : Outport  Port=2
  wires:
  Constant1/1 -> Efficiency/2
  financial costa/1 -> " financial cost yuan per kWh"/1
  Sc and Bat_Energy_useFul (Joule)1/1 -> Total energy consumption Bat+ Supercap (Joule)/2, Subtract/2
  Constant2/1 -> Subtract/1
  Constant3/1 -> Subtract1/1
  Divide2/1 -> Efficiency/1
  Total energy consumption Bat+ Supercap (Joule)/1 -> Gain2/1, Subtract1/2  "Joule to kWh"
  Efficiency/1 -> HESS_Efficiency/1
  Subtract1/1 -> Divide2/2
  Subtract/1 -> Divide1/1
  Gain2/1 -> financial costa/1
  Divide1/1 -> Divide2/1
  Bat_Energy_loss (Joule)/1 -> Total energy loss Bat+ Supercap/1
  SC_Energy_loss (Joule)1/1 -> Total energy loss Bat+ Supercap/2
  Total energy loss Bat+ Supercap/1 -> Total energy consumption Bat+ Supercap (Joule)/1
  yuan per kWh/1 -> financial costa/2
  SC_Energy_loss/1 -> SC_Energy_loss (Joule)1/1
  Sc and Bat_Energy_useFul/1 -> Sc and Bat_Energy_useFul (Joule)1/1
  "Bat_Energy_loss "/1 -> Bat_Energy_loss (Joule)/1

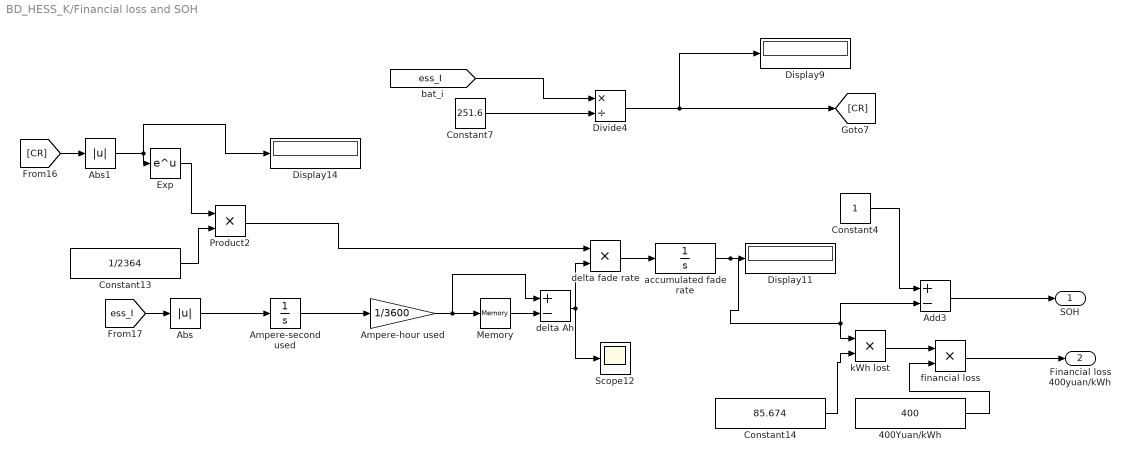
== system BD_HESS_K/Financial loss and SOH ==
  400Yuan/kWh : Constant  Value=400
  Abs : Abs  SaturateOnIntegerOverflow=off
  Abs1 : Abs  SaturateOnIntegerOverflow=off
  Add3 : Sum  Inputs=+-
  Ampere-hour used : Gain  Gain=1/3600
  Ampere-second used : Integrator
  Constant13 : Constant  Value=1/2364
  Constant14 : Constant  Value=85.674
  Constant4 : Constant
  Constant7 : Constant  Value=251.6
  Display11 : Display
  Display14 : Display
  Display9 : Display
  Divide4 : Product  Inputs=*/
  Exp : Math
  Memory : Memory
  Product2 : Product
  Scope12 : Scope
  accumulated fade rate : Integrator
  delta Ah : Sum  Inputs=+-
  delta fade rate : Product
  financial loss : Product
  kWh lost : Product
  SOH : Outport
  Financial loss 400yuan/kWh : Outport  Port=2
  wires:
  Add3/1 -> SOH/1
  kWh lost/1 -> financial loss/1
  Memory/1 -> delta Ah/2
  [ess_I] -> Abs/1
  delta fade rate/1 -> accumulated fade rate/1
  accumulated fade rate/1 -> kWh lost/1, Add3/2, Display11/1
  Abs1/1 -> Display14/1, Exp/1
  400Yuan/kWh/1 -> financial loss/2
  Divide4/1 -> Display9/1, [CR]
  Ampere-hour used/1 -> delta Ah/1, Memory/1
  Abs/1 -> Ampere-second used/1
  Product2/1 -> delta fade rate/1
  [CR] -> Abs1/1
  delta Ah/1 -> delta fade rate/2, Scope12/1
  [ess_I] -> Divide4/1
  Exp/1 -> Product2/1
  Constant7/1 -> Divide4/2
  Ampere-second used/1 -> Ampere-hour used/1
  Constant13/1 -> Product2/2
  Constant4/1 -> Add3/1
  Constant14/1 -> kWh lost/2
  financial loss/1 -> Financial loss 400yuan/kWh/1

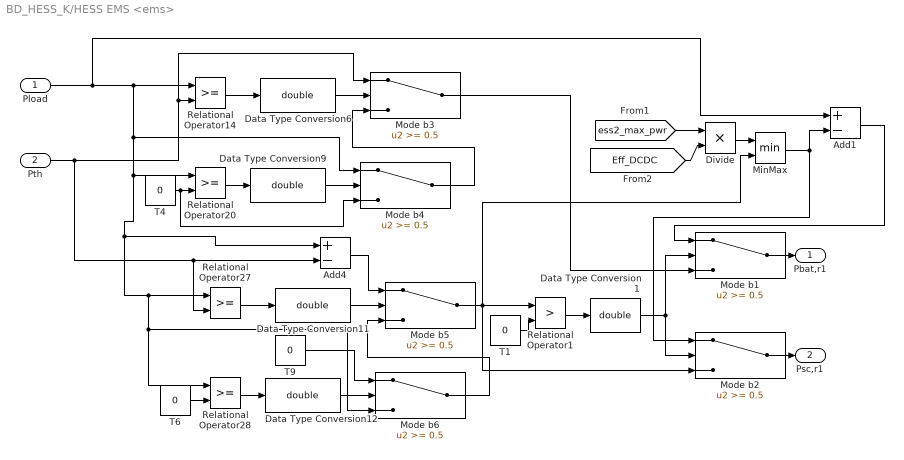
== system BD_HESS_K/HESS EMS <ems> ==
  Pload : Inport
  Pth : Inport  Port=2
  Add1 : Sum  Inputs=+-
  Add4 : Sum  Inputs=+-
  Data Type Conversion{1,6,9,11..12} (5 alike) : DataTypeConversion  OutDataTypeStr=double  SaturateOnIntegerOverflow=off  RndMeth=Floor
  Divide : Product  Inputs=**
  MinMax : MinMax  Inputs=2
  Mode b{1..6} (6 alike) : Switch  Threshold=0.5  SaturateOnIntegerOverflow=off  InputSameDT=off
  Relational Operator1 : RelationalOperator  Operator=>  OutDataTypeStr=boolean  InputSameDT=off
  Relational Operator{14,20,27..28} (4 alike) : RelationalOperator  OutDataTypeStr=boolean  InputSameDT=off
  T{1,4,6,9} (4 alike) : Constant  Value=0
  Pbat,r1 : Outport  PortDimensions=1  LockScale=on
  Psc,r1 : Outport  Port=2  PortDimensions=1
  wires:
  Relational Operator14/1 -> Data Type Conversion6/1
  Data Type Conversion6/1 -> Mode b3/2
  T4/1 -> Mode b4/3, Relational Operator20/2
  Data Type Conversion9/1 -> Mode b4/2
  Relational Operator20/1 -> Data Type Conversion9/1
  Mode b4/1 -> Mode b3/3
  Mode b6/1 -> Mode b5/3
  Data Type Conversion11/1 -> Mode b5/2
  Data Type Conversion12/1 -> Mode b6/2
  Relational Operator27/1 -> Data Type Conversion11/1
  Pload/1 -> Add1/1, Relational Operator14/1, Mode b4/1, Relational Operator27/1, Mode b6/3, Relational Operator28/1, Add4/1, Relational Operator20/1
  T6/1 -> Relational Operator28/2
  Pth/1 -> Add4/2, Relational Operator27/2, Mode b3/1, Relational Operator14/2
  Relational Operator28/1 -> Data Type Conversion12/1
  T9/1 -> Mode b6/1
  Add4/1 -> Mode b5/1
  T1/1 -> Relational Operator1/2
  Mode b5/1 -> MinMax/2, Relational Operator1/1, Mode b2/3
  Relational Operator1/1 -> Data Type Conversion1/1
  Mode b3/1 -> Mode b1/3
  Mode b1/1 -> Pbat,r1/1
  Mode b2/1 -> Psc,r1/1
  Data Type Conversion1/1 -> Mode b2/2, Mode b1/2
  [ess2_max_pwr] -> Divide/1
  [Eff_DCDC] -> Divide/2
  Divide/1 -> MinMax/1
  MinMax/1 -> Mode b2/1, Add1/2
  Add1/1 -> Mode b1/1

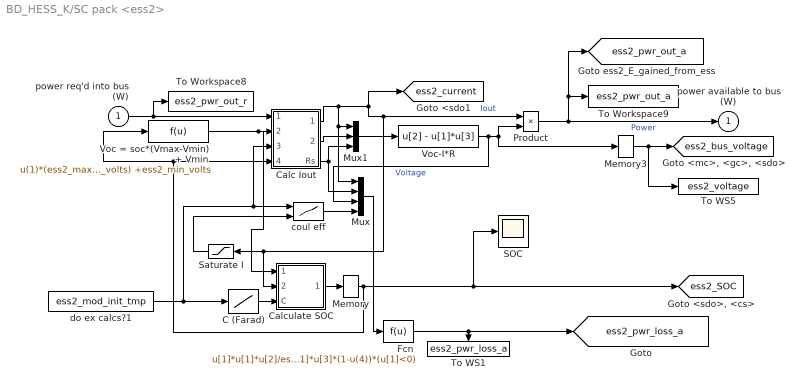
== system BD_HESS_K/SC pack <ess2>  ==
  power req'd into bus (W) : Inport
  C (Farad) : Lookup  InputValues=ess2_tmp  Table=ess2_cap
  Calc Iout : Subsystem
  Calculate SOC : Subsystem
  Fcn : Fcn  Expr=u[1]*u[1]*u[2]/ess2_parallel_mod_num*(u[1]>=0)+u[1]*u[1]*u(4)*u(4)*u[2]/ess2_parallel_mod_num*(u[1]<0)-u[1]*u[3]*(1-u(4))*(u[1]<0)
  Memory : Memory  InitialCondition=ess2_init_soc
  Memory3 : Memory  InitialCondition=(ess2_init_soc*(ess2_max_volts-ess2_min_volts) +ess2_min_volts)*ess2_module_num
  Mux : Mux
  Mux1 : Mux  Inputs=3
  Product : Product  InputSameDT=on  RndMeth=Zero  SaturateOnIntegerOverflow=on  OutDataTypeStr=Inherit: Same as first input
  SOC : Scope
  Saturate I : Saturate  UpperLimit=2600  LowerLimit=-2600
  To WS1 : ToWorkspace  VariableName=ess2_pwr_loss_a
  To WS5 : ToWorkspace  VariableName=ess2_voltage
  To Workspace8 : ToWorkspace  VariableName=ess2_pwr_out_r  SampleTime=-1
  To Workspace9 : ToWorkspace  VariableName=ess2_pwr_out_a  SampleTime=-1
  Voc = soc*(Vmax-Vmin) + Vmin : Fcn  Expr=u(1)*(ess2_max_volts-ess2_min_volts) +ess2_min_volts
  Voc-I*R : Fcn  Expr=u[2] - u[1]*u[3]
  coul eff : Lookup2D  RowIndex=ess2_tmp  ColumnIndex=ess2_i  Table=ess2_coulombic_eff
  do ex calcs?1 : Constant  Value=ess2_mod_init_tmp
  power available to bus (W) : Outport  InitialOutput=0
  tag scope: ess2_SOC=global, ess2_bus_voltage=global, ess2_current=global, ess2_pwr_loss_a=global, ess2_pwr_out_a=global
  wires:
  Calc Iout/2(Voc*k) -> Mux1/2
  Voc-I*R/1 -> Product/2, Memory3/1, Mux/3  "Voltage"
  Saturate I/1 -> coul eff/2
  Fcn/1 -> [ess2_pwr_loss_a], To WS1/1
  Mux/1 -> Fcn/1
  Product/1 -> power available to bus (W)/1, [ess2_pwr_out_a], To Workspace9/1  "Power"
  power req'd into bus (W)/1 -> Calc Iout/1(Preq), To Workspace8/1
  Memory3/1 -> [ess2_bus_voltage], To WS5/1
  Memory/1 -> SOC/1, [ess2_SOC], Voc = soc*(Vmax-Vmin) + Vmin/1, Calc Iout/4(SOC)
  Calculate SOC/1(SOC) -> Memory/1
  Calc Iout/1(Iout) -> Mux/1, Mux1/1, Product/1, Saturate I/1, Calculate SOC/2(Iout), [ess2_current]  "Iout"
  do ex calcs?1/1 -> C (Farad)/1, coul eff/1, Calc Iout/3(tmp)
  Voc = soc*(Vmax-Vmin) + Vmin/1 -> Calc Iout/2(Voc), Calculate SOC/1(Voc)
  C (Farad)/1 -> Calculate SOC/3(C)
  Mux1/1 -> Voc-I*R/1
  Calc Iout/3(Rs) -> Mux/2, Mux1/3
  coul eff/1 -> Mux/4

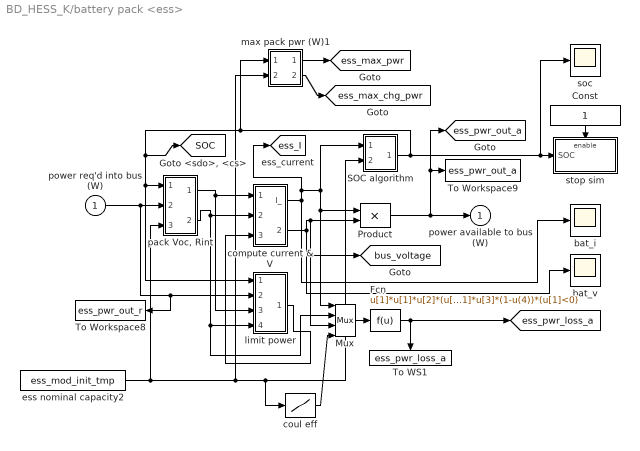
== system BD_HESS_K/battery pack <ess> ==
  power req'd into bus (W) : Inport
  " bat_i" : Scope
  " bat_v" : Scope
  Const : Constant
  Fcn : Fcn  Expr=u[1]*u[1]*u[2]*(u[1]>=0)+u[1]*u[1]*u[2]*u(4)*u(4)*(u[1]<0)-u[1]*u[3]*(1-u(4))*(u[1]<0)
  Mux : Mux
  Product : Product  InputSameDT=on  RndMeth=Zero  SaturateOnIntegerOverflow=on  OutDataTypeStr=Inherit: Same as first input
  SOC algorithm : Subsystem
  To WS1 : ToWorkspace  VariableName=ess_pwr_loss_a
  To Workspace8 : ToWorkspace  VariableName=ess_pwr_out_r  SampleTime=-1
  To Workspace9 : ToWorkspace  VariableName=ess_pwr_out_a  SampleTime=-1
  compute current & V : Subsystem
  coul eff : Lookup  InputValues=ess_tmp  Table=ess_coulombic_eff
  ess nominal capacity2 : Constant  Value=ess_mod_init_tmp
  "limit power " : Subsystem
  max pack pwr (W)1 : Subsystem
  "pack Voc, Rint" : Subsystem
  soc : Scope
  stop sim : Subsystem  TreatAsAtomicUnit=on
  power available to bus (W) : Outport  InitialOutput=0
  tag scope: SOC=global, bus_voltage=global, ess_I=global, ess_max_chg_pwr=global, ess_max_pwr=global, ess_pwr_loss_a=global, ess_pwr_out_a=global
  wires:
  max pack pwr (W)1/2(max ess charge pwr) -> [ess_max_chg_pwr]
  ess nominal capacity2/1 -> SOC algorithm/2(tmp (C)), coul eff/1, max pack pwr (W)1/2(ess_mod_tmp), "pack Voc, Rint"/3(mod tmp (C))
  max pack pwr (W)1/1(max ess discharge pwr) -> [ess_max_pwr]
  coul eff/1 -> Mux/4
  "limit power "/1("Pbty, limited") -> compute current & V/3(limited output power (W))
  "pack Voc, Rint"/1(pack open- circuit voltage) -> "limit power "/3(Voc), compute current & V/1(Voc)
  "pack Voc, Rint"/2(pack resistance) -> Mux/2, "limit power "/4(Rint), compute current & V/2(Rint)
  Const/1 -> stop sim/Enable
  SOC algorithm/1(SOC1) -> max pack pwr (W)1/1(SOC), "limit power "/1(SOC), "pack Voc, Rint"/1(SOC (prev)), [SOC], soc/1, stop sim/1(SOC)
  Fcn/1 -> To WS1/1, [ess_pwr_loss_a]
  Product/1 -> [ess_pwr_out_a], To Workspace9/1, power available to bus (W)/1
  compute current & V/1(I_) -> [ess_I], Mux/1, Product/1, SOC algorithm/1((A)), " bat_i"/1
  power req'd into bus (W)/1 -> "pack Voc, Rint"/2(req'd battery power (W)), "limit power "/2(Pbty), To Workspace8/1
  Mux/1 -> Fcn/1
  compute current & V/2(V_) -> [bus_voltage], Mux/3, Product/2, " bat_v"/1

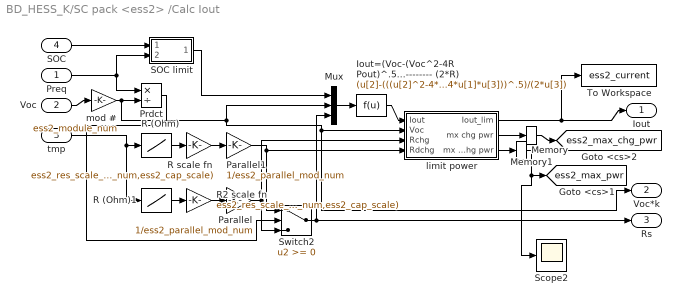
== system BD_HESS_K/SC pack <ess2> /Calc Iout ==
  Preq : Inport
  Voc : Inport  Port=2
  tmp : Inport  Port=3
  SOC : Inport  Port=4
  Iout=(Voc-(Voc^2-4RPout)^.5) ----------------------------- (2*R) : Fcn  Expr=(u[2]-(((u[2]^2-4*u[1]*u[3])>0)*(u[2]^2-4*u[1]*u[3]))^.5)/(2*u[3])
  Memory : Memory
  Memory1 : Memory
  Mux : Mux  Inputs=3
  Parallel : Gain  Gain=1/ess2_parallel_mod_num  SaturateOnIntegerOverflow=on  OutDataTypeStr=Inherit: Same as input  ParamDataTypeStr=Inherit: Same as input
  Parallel1 : Gain  Gain=1/ess2_parallel_mod_num  SaturateOnIntegerOverflow=on  OutDataTypeStr=Inherit: Same as input  ParamDataTypeStr=Inherit: Same as input
  Prdct : Product  Inputs=*/  InputSameDT=on  RndMeth=Zero  SaturateOnIntegerOverflow=on  OutDataTypeStr=Inherit: Same as first input
  R (Ohm) : Lookup  InputValues=ess2_tmp  Table=ess2_r
  R (Ohm)1 : Lookup  InputValues=ess2_tmp  Table=ess2_r
  R scale fn : Gain  Gain=ess2_res_scale_fun(ess2_res_scale_coef,ess2_module_num,ess2_cap_scale)  SaturateOnIntegerOverflow=on  OutDataTypeStr=Inherit: Same as input  ParamDataTypeStr=Inherit: Same as input
  R2 scale fn : Gain  Gain=ess2_res_scale_fun(ess2_res_scale_coef,ess2_module_num,ess2_cap_scale)  SaturateOnIntegerOverflow=on  OutDataTypeStr=Inherit: Same as input  ParamDataTypeStr=Inherit: Same as input
  SOC limit : Subsystem
  Scope2 : Scope
  Switch2 : Switch
  To Workspace : ToWorkspace  VariableName=ess2_current  SampleTime=-1
  limit power : Subsystem
  mod # : Gain  Gain=ess2_module_num  SaturateOnIntegerOverflow=on  OutDataTypeStr=Inherit: Same as input  ParamDataTypeStr=Inherit: Same as input
  Iout : Outport
  Voc*k : Outport  Port=2
  Rs : Outport  Port=3
  tag scope: ess2_max_chg_pwr=global, ess2_max_pwr=global
  wires:
  Preq/1 -> Prdct/1, SOC limit/2(Pbty)
  SOC/1 -> SOC limit/1(SOC)
  Mux/1 -> Iout=(Voc-(Voc^2-4RPout)^.5) ----------------------------- (2*R)/1
  R (Ohm)/1 -> R scale fn/1
  R scale fn/1 -> Parallel1/1
  R (Ohm)1/1 -> R2 scale fn/1
  Prdct/1 -> Switch2/2
  R2 scale fn/1 -> Parallel/1
  SOC limit/1("Pbty, limited") -> Mux/1
  Switch2/1 -> Rs/1, Mux/3
  limit power/1(Iout_lim) -> Iout/1, To Workspace/1
  Iout=(Voc-(Voc^2-4RPout)^.5) ----------------------------- (2*R)/1 -> limit power/1(Iout)
  Voc/1 -> mod #/1
  mod #/1 -> Mux/2, limit power/2(Voc), Voc*k/1, Prdct/2
  tmp/1 -> R (Ohm)1/1, R (Ohm)/1
  Memory/1 -> Scope2/1, [ess2_max_pwr]
  limit power/3(mx dchg pwr) -> Memory/1
  limit power/2(mx chg pwr) -> Memory1/1
  Memory1/1 -> [ess2_max_chg_pwr]
  Parallel1/1 -> Switch2/1, limit power/4(Rdchg)
  Parallel/1 -> Switch2/3, limit power/3(Rchg)

== system BD_HESS_K/SC pack <ess2> /Calculate SOC ==
  Voc : Inport
  Iout : Inport  Port=2
  C : Inport  Port=3
  Clock : Clock
  Gain : Gain  Gain=ess2_parallel_mod_num  SaturateOnIntegerOverflow=on  OutDataTypeStr=Inherit: Same as input  ParamDataTypeStr=Inherit: Same as input
  Memory : Memory
  Mux1 : Mux
  Saturation : Saturate  UpperLimit=1  LowerLimit=0
  Soc = (Voc(n+1)-Vmin)/(Vmax-Vmin) : Fcn  Expr=(u(1)-ess2_min_volts)/(ess2_max_volts-ess2_min_volts)
  Sum : Sum  Inputs=|+-  InputSameDT=on  SaturateOnIntegerOverflow=on  OutDataTypeStr=Inherit: Same as first input
  Voc (n+1) = Voc(n) - I*(dt)/C : Fcn  Expr=(u(1) - u(2)*u(4)/u(3))
  SOC : Outport
  wires:
  Voc/1 -> Mux1/1
  Mux1/1 -> Voc (n+1) = Voc(n) - I*(dt)/C/1
  Iout/1 -> Mux1/2
  Voc (n+1) = Voc(n) - I*(dt)/C/1 -> Soc = (Voc(n+1)-Vmin)/(Vmax-Vmin)/1
  C/1 -> Gain/1
  Soc = (Voc(n+1)-Vmin)/(Vmax-Vmin)/1 -> Saturation/1
  Memory/1 -> Sum/2
  Clock/1 -> Memory/1, Sum/1
  Sum/1 -> Mux1/4
  Saturation/1 -> SOC/1
  Gain/1 -> Mux1/3

== system BD_HESS_K/battery pack <ess>/SOC algorithm ==
  note: SOC=(Max Ah capacity-Ah used)/Max Ah capacity
  (A) : Inport
  tmp (C) : Inport  Port=2
  (sec->hrs) : Gain  Gain=1/3600  SaturateOnIntegerOverflow=on  OutDataTypeStr=Inherit: Same as input  ParamDataTypeStr=Inherit: Same as input
  0 <= SOC <= 1 : Saturate  UpperLimit=1  LowerLimit=0
  A-h remaining : Sum  Inputs=-+  InputSameDT=on  SaturateOnIntegerOverflow=on  OutDataTypeStr=Inherit: Same as first input
  Ah used : Integrator  InitialConditionSource=external  InitialCondition=(1-ess_init_soc)*ess_max_ah_cap
  Fcn : Fcn  Expr=1/u
  Fcn1 : Fcn  Expr=(1-ess_init_soc)*u[1]
  SOC : Product  InputSameDT=on  RndMeth=Zero  SaturateOnIntegerOverflow=on  OutDataTypeStr=Inherit: Same as first input
  Switch : Switch
  adjusted A : Product  InputSameDT=on  RndMeth=Zero  SaturateOnIntegerOverflow=on  OutDataTypeStr=Inherit: Same as first input
  coul eff : Lookup  InputValues=ess_tmp  Table=ess_coulombic_eff
  max cap : Lookup  InputValues=ess_tmp  Table=ess_max_ah_cap*ess_cap_scale
  SOC1 : Outport  InitialOutput=0
  wires:
  (A)/1 -> Switch/2, Switch/1, adjusted A/1
  Switch/1 -> (sec->hrs)/1
  (sec->hrs)/1 -> Ah used/1
  Ah used/1 -> A-h remaining/1
  Fcn/1 -> SOC/2
  SOC/1 -> 0 <= SOC <= 1/1
  A-h remaining/1 -> SOC/1
  0 <= SOC <= 1/1 -> SOC1/1
  tmp (C)/1 -> max cap/1, coul eff/1
  coul eff/1 -> adjusted A/2
  adjusted A/1 -> Switch/3
  max cap/1 -> A-h remaining/2, Fcn/1, Fcn1/1
  Fcn1/1 -> Ah used/2

== system BD_HESS_K/battery pack <ess>/compute current & V ==
  Voc : Inport
  Rint : Inport  Port=2
  limited output power (W) : Inport  Port=3
  Ibty=(Voc-(Voc^2-4RPbty)^.5) ----------------------------- (2*R) : Fcn  Expr=(u[2]-(u[2]^2-4*u[1]*u[3])^.5)/(2*u[3])
  Logical Operator1 : Logic  Operator=NOT  Inputs=1
  Mux3 : Mux  Inputs=3
  Mux4 : Mux  Inputs=3
  Mux5 : Mux  Inputs=3
  To Workspace9 : ToWorkspace  VariableName=ess_current  SampleTime=-1
  Voc-I*R : Fcn  Expr=u[2]-u[1]*u[3]
  ess max voltage*#batts : Constant  Value=ess_max_volts*ess_module_num
  iabs min=(Voc-Vmax)/R max_charging_current : Fcn  Expr=(u(1)-u(2))/u(3)
  limit current based on max voltage during charge : Switch  Threshold=eps
  min charge current not exceeded : RelationalOperator  Operator=>
  I_ : Outport  InitialOutput=0
  V_ : Outport  Port=2  InitialOutput=0
  tag scope: ess_maxV_limited=global
  wires:
  limited output power (W)/1 -> Mux4/1
  Voc/1 -> Mux4/2, Mux3/2, Mux5/1
  Rint/1 -> Mux4/3, Mux3/3, Mux5/3
  Ibty=(Voc-(Voc^2-4RPbty)^.5) ----------------------------- (2*R)/1 -> min charge current not exceeded/1, limit current based on max voltage during charge/1
  iabs min=(Voc-Vmax)/R max_charging_current/1 -> min charge current not exceeded/2, limit current based on max voltage during charge/3
  limit current based on max voltage during charge/1 -> I_/1, To Workspace9/1, Mux3/1
  min charge current not exceeded/1 -> limit current based on max voltage during charge/2, Logical Operator1/1
  Mux3/1 -> Voc-I*R/1
  Voc-I*R/1 -> V_/1
  Mux4/1 -> Ibty=(Voc-(Voc^2-4RPbty)^.5) ----------------------------- (2*R)/1
  Mux5/1 -> iabs min=(Voc-Vmax)/R max_charging_current/1
  ess max voltage*#batts/1 -> Mux5/2
  Logical Operator1/1 -> [ess_maxV_limited]

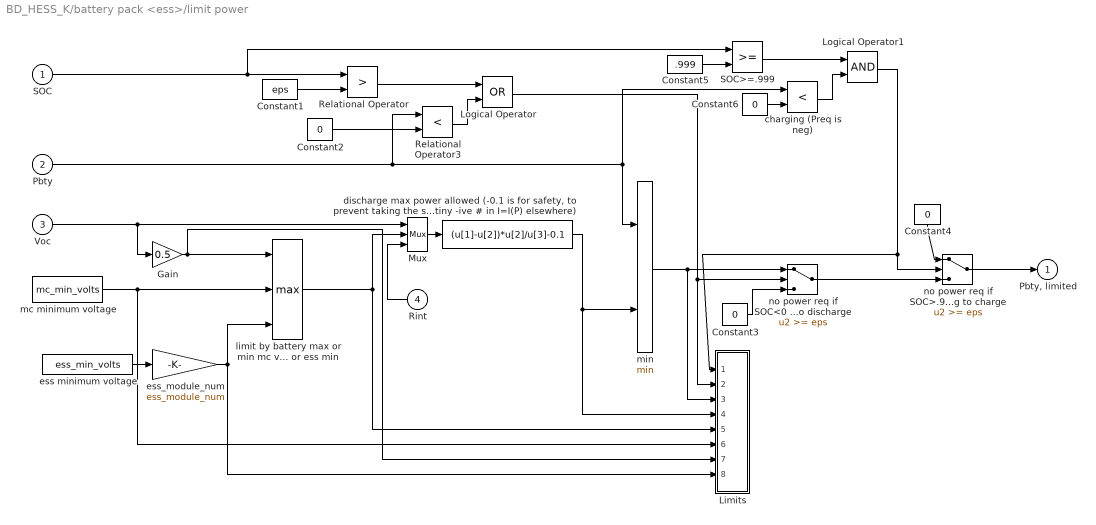
== system BD_HESS_K/battery pack <ess>/limit power  ==
  SOC : Inport
  Pbty : Inport  Port=2
  Voc : Inport  Port=3
  Rint : Inport  Port=4
  Constant1 : Constant  Value=eps
  Constant{2..4,6} (4 alike) : Constant  Value=0
  Constant5 : Constant  Value=.999
  Gain : Gain  Gain=0.5  SaturateOnIntegerOverflow=on  OutDataTypeStr=Inherit: Same as input  ParamDataTypeStr=Inherit: Same as input
  Limits : Subsystem
  Logical Operator : Logic  Operator=OR
  Logical Operator1 : Logic
  Mux : Mux  Inputs=3
  Relational Operator : RelationalOperator  Operator=>
  Relational Operator3 : RelationalOperator  Operator=<
  SOC>=.999 : RelationalOperator
  charging (Preq is neg) : RelationalOperator  Operator=<
  "discharge max power allowed (-0.1 is for safety, to prevent taking the square of a tiny -ive # in I=I(P) elsewhere)" : Fcn  Expr=(u[1]-u[2])*u[2]/u[3]-0.1
  ess minimum voltage : Constant  Value=ess_min_volts
  ess_module_num : Gain  Gain=ess_module_num  SaturateOnIntegerOverflow=on  OutDataTypeStr=Inherit: Same as input  ParamDataTypeStr=Inherit: Same as input
  limit by battery max or min mc voltage or ess min : MinMax  Function=max  Inputs=3  InputSameDT=on  SaturateOnIntegerOverflow=on
  mc minimum voltage : Constant  Value=mc_min_volts
  min : MinMax  Inputs=2  InputSameDT=on  SaturateOnIntegerOverflow=on
  no power req if SOC<0 and trying to discharge : Switch  Threshold=eps
  no power req if SOC>.999 and trying to charge : Switch  Threshold=eps
  "Pbty, limited" : Outport  InitialOutput=0
  wires:
  Constant1/1 -> Relational Operator/2
  Relational Operator/1 -> Logical Operator/1
  Pbty/1 -> Relational Operator3/1, min/1, charging (Preq is neg)/1
  Constant2/1 -> Relational Operator3/2
  Relational Operator3/1 -> Logical Operator/2
  Constant3/1 -> no power req if SOC<0 and trying to discharge/3
  Logical Operator/1 -> no power req if SOC<0 and trying to discharge/2, Limits/2(not SOC low limited)
  Voc/1 -> Mux/1, Gain/1
  min/1 -> no power req if SOC<0 and trying to discharge/1, Limits/3(power req)
  Mux/1 -> "discharge max power allowed (-0.1 is for safety, to prevent taking the square of a tiny -ive # in I=I(P) elsewhere)"/1
  limit by battery max or min mc voltage or ess min/1 -> Mux/2, Limits/5(V used)
  "discharge max power allowed (-0.1 is for safety, to prevent taking the square of a tiny -ive # in I=I(P) elsewhere)"/1 -> Limits/4(power bat limited), min/2
  mc minimum voltage/1 -> limit by battery max or min mc voltage or ess min/2, Limits/6(V mc_min_volts)
  Rint/1 -> Mux/3
  Gain/1 -> limit by battery max or min mc voltage or ess min/1, Limits/7(V battery (.5Voc))
  ess minimum voltage/1 -> ess_module_num/1
  ess_module_num/1 -> limit by battery max or min mc voltage or ess min/3, Limits/8(V ess_min_volts)
  SOC/1 -> Relational Operator/1, SOC>=.999/1
  SOC>=.999/1 -> Logical Operator1/1
  Constant6/1 -> charging (Preq is neg)/2
  charging (Preq is neg)/1 -> Logical Operator1/2
  Constant5/1 -> SOC>=.999/2
  Constant4/1 -> no power req if SOC>.999 and trying to charge/1
  no power req if SOC<0 and trying to discharge/1 -> no power req if SOC>.999 and trying to charge/3
  no power req if SOC>.999 and trying to charge/1 -> "Pbty, limited"/1
  Logical Operator1/1 -> no power req if SOC>.999 and trying to charge/2, Limits/1(SOC high limited)

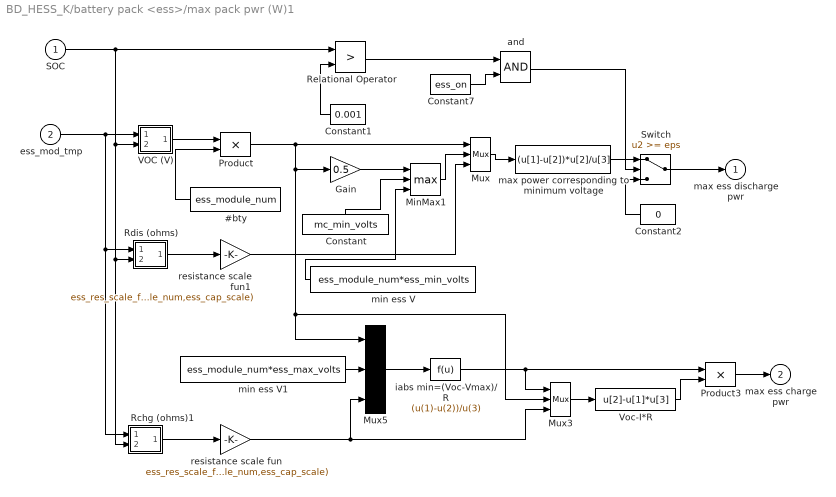
== system BD_HESS_K/battery pack <ess>/max pack pwr (W)1 ==
  SOC : Inport
  ess_mod_tmp : Inport  Port=2
  #bty : Constant  Value=ess_module_num
  Constant : Constant  Value=mc_min_volts
  Constant1 : Constant  Value=0.001
  Constant2 : Constant  Value=0
  Constant7 : Constant  Value=ess_on
  Gain : Gain  Gain=0.5  SaturateOnIntegerOverflow=on  OutDataTypeStr=Inherit: Same as input  ParamDataTypeStr=Inherit: Same as input
  MinMax1 : MinMax  Function=max  Inputs=3  InputSameDT=on  SaturateOnIntegerOverflow=on
  Mux : Mux  Inputs=3
  Mux3 : Mux  Inputs=3
  Mux5 : Mux  Inputs=3
  Product : Product  InputSameDT=on  RndMeth=Zero  SaturateOnIntegerOverflow=on  OutDataTypeStr=Inherit: Same as first input
  Product3 : Product  InputSameDT=on  RndMeth=Zero  SaturateOnIntegerOverflow=on  OutDataTypeStr=Inherit: Same as first input
  Rchg (ohms)1 : Subsystem  mask(2-D Table Lookup){xindex=ess_tmp, yindex=ess_soc, table=ess_r_chg}
      mask prompts: xindex "X Index"; yindex "Y Index"
      mask help:
      | Two Dimensional Table Lookup
      | The first input corresponds to X Index and the second input corresponds to the Y Index
      mask init:
      | sftab2chk(xindex,yindex,table);
      mask Help: This block returns a linearly interpolated intersection from the table using the X index (which corresponds to the rows of the table) and the Y index (which corresponds to the columns of the table).  Extrapolation is used.
      mask Display: plot(-10,-10,110,110,[90,50,10],[90,40,30],[90,50,10],[50,26,20],[90,50,10],[22,13,10])
  Rdis (ohms) : Subsystem  mask(2-D Table Lookup){xindex=ess_tmp, yindex=ess_soc, table=ess_r_dis}
      mask prompts: xindex "X Index"; yindex "Y Index"
      mask help:
      | Two Dimensional Table Lookup
      | The first input corresponds to X Index and the second input corresponds to the Y Index
      mask init:
      | sftab2chk(xindex,yindex,table);
      mask Help: This block returns a linearly interpolated intersection from the table using the X index (which corresponds to the rows of the table) and the Y index (which corresponds to the columns of the table).  Extrapolation is used.
      mask Display: plot(-10,-10,110,110,[90,50,10],[90,40,30],[90,50,10],[50,26,20],[90,50,10],[22,13,10])
  Relational Operator : RelationalOperator  Operator=>
  Switch : Switch  Threshold=eps
  VOC (V) : Subsystem  mask(2-D Table Lookup){xindex=ess_tmp, yindex=ess_soc, table=ess_voc}
      mask prompts: xindex "X Index"; yindex "Y Index"
      mask help:
      | Two Dimensional Table Lookup
      | The first input corresponds to X Index and the second input corresponds to the Y Index
      mask init:
      | sftab2chk(xindex,yindex,table);
      mask Help: This block returns a linearly interpolated intersection from the table using the X index (which corresponds to the rows of the table) and the Y index (which corresponds to the columns of the table).  Extrapolation is used.
      mask Display: plot(-10,-10,110,110,[90,50,10],[90,40,30],[90,50,10],[50,26,20],[90,50,10],[22,13,10])
  Voc-I*R : Fcn  Expr=u[2]-u[1]*u[3]
  and : Logic
  iabs min=(Voc-Vmax)/R : Fcn  Expr=(u(1)-u(2))/u(3)
  max power corresponding to minimum voltage : Fcn  Expr=(u[1]-u[2])*u[2]/u[3]
  min ess V : Constant  Value=ess_module_num*ess_min_volts
  min ess V1 : Constant  Value=ess_module_num*ess_max_volts
  resistance scale fun : Gain  Gain=ess_res_scale_fun(ess_res_scale_coef,ess_module_num,ess_cap_scale)  SaturateOnIntegerOverflow=on  OutDataTypeStr=Inherit: Same as input  ParamDataTypeStr=Inherit: Same as input
  resistance scale fun1 : Gain  Gain=ess_res_scale_fun(ess_res_scale_coef,ess_module_num,ess_cap_scale)  SaturateOnIntegerOverflow=on  OutDataTypeStr=Inherit: Same as input  ParamDataTypeStr=Inherit: Same as input
  max ess discharge pwr : Outport  InitialOutput=0
  max ess charge pwr : Outport  Port=2  InitialOutput=0
  wires:
  #bty/1 -> Product/2
  Rchg (ohms)1/1(table out) -> resistance scale fun/1
  resistance scale fun/1 -> Mux3/3, Mux5/3
  Product3/1 -> max ess charge pwr/1
  Voc-I*R/1 -> Product3/2
  iabs min=(Voc-Vmax)/R/1 -> Product3/1, Mux3/1
  Mux3/1 -> Voc-I*R/1
  Mux5/1 -> iabs min=(Voc-Vmax)/R/1
  min ess V1/1 -> Mux5/2
  Switch/1 -> max ess discharge pwr/1
  SOC/1 -> Rchg (ohms)1/2(y0), Rdis (ohms)/2(y0), VOC (V)/2(y0), Relational Operator/1
  Constant2/1 -> Switch/3
  max power corresponding to minimum voltage/1 -> Switch/1
  Rdis (ohms)/1(table out) -> resistance scale fun1/1
  VOC (V)/1(table out) -> Product/1
  resistance scale fun1/1 -> Mux/3
  Product/1 -> Mux3/2, Mux5/1, Gain/1, Mux/1
  MinMax1/1 -> Mux/2
  Gain/1 -> MinMax1/1
  Mux/1 -> max power corresponding to minimum voltage/1
  Constant/1 -> MinMax1/2
  Constant1/1 -> Relational Operator/2
  ess_mod_tmp/1 -> Rchg (ohms)1/1(x0), Rdis (ohms)/1(x0), VOC (V)/1(x0)
  min ess V/1 -> MinMax1/3
  and/1 -> Switch/2
  Relational Operator/1 -> and/1
  Constant7/1 -> and/2
